simulink model "basic_2"  (R2023b)
settings: Solver=VariableStepAuto  StartTime=0.0  StopTime=10.0  RelTol=1e-3
settings Model: Creator=simon  LastModifiedBy=simon

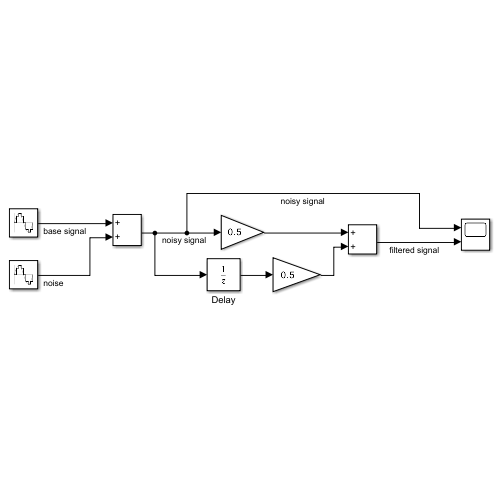
[thumbnail: Simulink's stored preview of the top-level diagram]
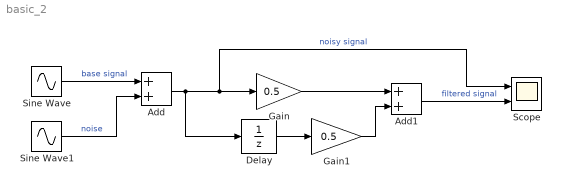
== system basic_2 ==
  Add : Sum
  Add1 : Sum
  Delay : UnitDelay  SampleTime=.2  HasFrameUpgradeWarning=on
  Gain : Gain  Gain=0.5
  Gain1 : Gain  Gain=0.5
  Scope : Scope  NumInputPorts=2
  Sine Wave : Sin  Amplitude=10  SampleTime=.2
  Sine Wave1 : Sin  Amplitude=2.5  Frequency=18  SampleTime=.2
  wires:
  Gain/1 -> Add1/1
  Sine Wave/1 -> Add/1  "base signal"
  Add/1 -> Scope/1, Gain/1, Delay/1  "noisy signal"
  Delay/1 -> Gain1/1
  Sine Wave1/1 -> Add/2  "noise"
  Gain1/1 -> Add1/2
  Add1/1 -> Scope/2  "filtered signal"
